simulink model "APFC_FullModel_v23_NoALPF_NodqLPF"  (R2025b)
settings: Solver=ode23t  StartTime=0.0  StopTime=50  MaxStep=2e-4  RelTol=1e-3
undefined symbols (not defined in the file): ALPF_fs, C_B1, C_B2, C_B3, DiscIntNeverNeededParam, FLC_deadband_kVAR, L_B1, L_B2, L_B3, omega, p, Q_reactor, Rc, tau_Qload, X1
libraries: ee_lib x63, fl_lib x59, nesl_utility x43, dspswit3 x9, eeTransforms x2, fuzblock x1, eeSinusoidalMeasurementV2 x1
(part 2 of 4)

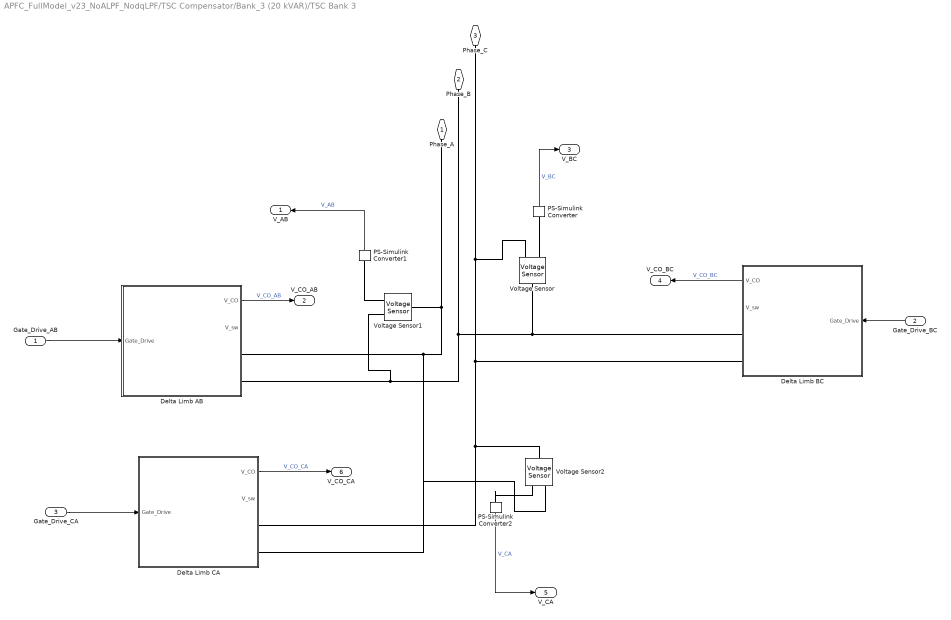
== system APFC_FullModel_v23_NoALPF_NodqLPF/TSC Compensator/Bank_3 (20 kVAR)/TSC Bank 3 ==
  Gate_Drive_AB : Inport
  Gate_Drive_BC : Inport  Port=2
  Gate_Drive_CA : Inport  Port=3
  Delta Limb AB : Subsystem  mask{C_val=C_B3, L_val=L_B3, Rd_val=100e3}
      mask prompts: C_val "Capacitance (F)"; L_val "Inductance (H)"; Rd_val "Discharge Resistance (Ohm)"
      mask help:
      | Delta limb of a three-phase delta-connected TSC bank.
      | Contains: anti-parallel thyristor pair, detuning reactor (L_val,
      | R_series = omega*L_val/Q_reactor), shunt capacitor (C_val), parallel discharge
      | resistor (Rd_val), RC snubber (100 Ohm, 0.1 uF).
      |
      | Output signals:
      | V_sw: instantaneous voltage across the anti-parallel thyristor pair.
      | Used as a diagnostic signal to verify transient-free switching.
      | At the moment of firing, V_sw should be at or near zero. After
      | turn-off, V_sw reflects the difference between the line-to-line
      | source voltage and the capacitor voltage V_C0.
      |
      | V_C0: instantaneous voltage across the shunt capacitor. Fed
      | externally to the ZCD comparator as the residual capacitor voltage
      | reference for voltage-matched firing on subsequent switching events.
      |
      | ZCD logic and gate drive signals are external to this subsystem.
      | Default values correspond to Bank 3 (20 kVAR) at 415 V / 50 Hz
      | with 6% detuning factor. Parameter values for Bank 1 (5 kVAR) and
      | Bank 2 (10 kVAR) are assigned by editing the mask dialog at
      | instantiation.
  Delta Limb BC : Subsystem  mask{C_val=C_B3, L_val=L_B3, Rd_val=100e3}
      mask prompts: C_val "Capacitance (F)"; L_val "Inductance (H)"; Rd_val "Discharge Resistance (Ohm)"
      mask help:
      | Delta limb of a three-phase delta-connected TSC bank.
      | Contains: anti-parallel thyristor pair, detuning reactor (L_val,
      | R_series = omega*L_val/Q_reactor), shunt capacitor (C_val), parallel discharge
      | resistor (Rd_val), RC snubber (100 Ohm, 0.1 uF).
      |
      | Output signals:
      | V_sw: instantaneous voltage across the anti-parallel thyristor pair.
      | Used as a diagnostic signal to verify transient-free switching.
      | At the moment of firing, V_sw should be at or near zero. After
      | turn-off, V_sw reflects the difference between the line-to-line
      | source voltage and the capacitor voltage V_C0.
      |
      | V_C0: instantaneous voltage across the shunt capacitor. Fed
      | externally to the ZCD comparator as the residual capacitor voltage
      | reference for voltage-matched firing on subsequent switching events.
      |
      | ZCD logic and gate drive signals are external to this subsystem.
      | Default values correspond to Bank 3 (20 kVAR) at 415 V / 50 Hz
      | with 6% detuning factor. Parameter values for Bank 1 (5 kVAR) and
      | Bank 2 (10 kVAR) are assigned by editing the mask dialog at
      | instantiation.
  Delta Limb CA : Subsystem  mask{C_val=C_B3, L_val=L_B3, Rd_val=100e3}
      mask prompts: C_val "Capacitance (F)"; L_val "Inductance (H)"; Rd_val "Discharge Resistance (Ohm)"
      mask help:
      | Delta limb of a three-phase delta-connected TSC bank.
      | Contains: anti-parallel thyristor pair, detuning reactor (L_val,
      | R_series = omega*L_val/Q_reactor), shunt capacitor (C_val), parallel discharge
      | resistor (Rd_val), RC snubber (100 Ohm, 0.1 uF).
      |
      | Output signals:
      | V_sw: instantaneous voltage across the anti-parallel thyristor pair.
      | Used as a diagnostic signal to verify transient-free switching.
      | At the moment of firing, V_sw should be at or near zero. After
      | turn-off, V_sw reflects the difference between the line-to-line
      | source voltage and the capacitor voltage V_C0.
      |
      | V_C0: instantaneous voltage across the shunt capacitor. Fed
      | externally to the ZCD comparator as the residual capacitor voltage
      | reference for voltage-matched firing on subsequent switching events.
      |
      | ZCD logic and gate drive signals are external to this subsystem.
      | Default values correspond to Bank 3 (20 kVAR) at 415 V / 50 Hz
      | with 6% detuning factor. Parameter values for Bank 1 (5 kVAR) and
      | Bank 2 (10 kVAR) are assigned by editing the mask dialog at
      | instantiation.
  PS-Simulink Converter : nesl_utility/PS-Simulink Converter  PhysicalDomain=network_engine_domain  SubClassName=ps_output  LeftPortType=input  RightPortType=output  PseudoPeriodic=off  Frequencies=[]  VectorFormat=inherit  Unit=inherit  AffineConversion=off
  PS-Simulink Converter1 : nesl_utility/PS-Simulink Converter  PhysicalDomain=network_engine_domain  SubClassName=ps_output  LeftPortType=input  RightPortType=output  PseudoPeriodic=off  Frequencies=[]  VectorFormat=inherit  Unit=inherit  AffineConversion=off
  PS-Simulink Converter2 : nesl_utility/PS-Simulink Converter  PhysicalDomain=network_engine_domain  SubClassName=ps_output  LeftPortType=input  RightPortType=output  PseudoPeriodic=off  Frequencies=[]  VectorFormat=inherit  Unit=inherit  AffineConversion=off
  Voltage Sensor : fl_lib/Electrical/Electrical Sensors/Voltage Sensor
  Voltage Sensor1 : fl_lib/Electrical/Electrical Sensors/Voltage Sensor
  Voltage Sensor2 : fl_lib/Electrical/Electrical Sensors/Voltage Sensor
  Phase_A : PMIOPort  Side=Left
  Phase_B : PMIOPort  Port=2  Side=Left
  Phase_C : PMIOPort  Port=3  Side=Left
  V_AB : Outport
  V_CO_AB : Outport  Port=2
  V_BC : Outport  Port=3
  V_CO_BC : Outport  Port=4
  V_CA : Outport  Port=5
  V_CO_CA : Outport  Port=6
  wires:
  Delta Limb BC/1(V_CO) -> V_CO_BC/1  "V_CO_BC"
  PS-Simulink Converter/1 -> V_BC/1  "V_BC"
  Gate_Drive_CA/1 -> Delta Limb CA/1(Gate_Drive)
  PS-Simulink Converter1/1 -> V_AB/1  "V_AB"
  Delta Limb AB/1(V_CO) -> V_CO_AB/1  "V_CO_AB"
  Delta Limb CA/1(V_CO) -> V_CO_CA/1  "V_CO_CA"
  Gate_Drive_BC/1 -> Delta Limb BC/1(Gate_Drive)
  Gate_Drive_AB/1 -> Delta Limb AB/1(Gate_Drive)
  PS-Simulink Converter2/1 -> V_CA/1  "V_CA"
  connections:
  Delta Limb BC/RConn1 -- Voltage Sensor/LConn1 -- Phase_B/RConn1 -- Voltage Sensor1/RConn2 -- Delta Limb AB/RConn2
  Voltage Sensor1/RConn1 -- PS-Simulink Converter1/LConn1
  PS-Simulink Converter2/LConn1 -- Voltage Sensor2/RConn1
  Voltage Sensor/RConn2 -- Phase_C/RConn1 -- Delta Limb BC/RConn2 -- Voltage Sensor2/LConn1 -- Delta Limb CA/RConn1
  Voltage Sensor/RConn1 -- PS-Simulink Converter/LConn1
  Voltage Sensor1/LConn1 -- Phase_A/RConn1 -- Voltage Sensor2/RConn2 -- Delta Limb CA/RConn2 -- Delta Limb AB/RConn1

== system APFC_FullModel_v23_NoALPF_NodqLPF/TSC Compensator/Bank_3 (20 kVAR)/ZCD Bank 3 ==
  V_AB : Inport
  V_CO_AB : Inport  Port=2
  V_BC : Inport  Port=3
  V_CO_BC : Inport  Port=4
  V_CA : Inport  Port=5
  V_CO_CA : Inport  Port=6
  Enable : Inport  Port=7
  ZCD AB : Subsystem
      mask help:
      | Zero-Crossing Detection (ZCD) subsystem for one delta limb of a
      | three-phase delta-connected TSC bank.
      |
      | Implements voltage-matched firing logic for transient-free
      | thyristor switching.
      |
      | Inputs:
      | V_source: instantaneous line-to-line voltage for this limb,
      | fed through a Unit Delay (T_s = 0.0001 s) to the comparator.
      |
      | V_C0: residual capacitor voltage from the corresponding
      | Delta_Limb instance, fed through a Unit Delay (T_s = 0.0001 s)
      | to the comparator.
      |
      | Enable: FLC switching command (S = 1 to arm, S = 0 to inhibit).
      | Set to Constant = 1 for open-loop testing.
      |
      | Output:
      | Gate_drive: firing pulse issued when V_source >= V_C0 on a
      | rising edge, AND Enable = 1. Fed to the Gate_drive inport of
      | the corresponding Delta_Limb instance.
      |
      | Internal blocks: Unit Delay (x2), Relational Operator (>=),
      | Zero-Order Hold (T_s = 0.0001 s), Edge Detector (rising edge),
      | AND gate.
      |
      | One instance required per delta limb: ZCD_AB, ZCD_BC, ZCD_CA.
  ZCD BC : Subsystem
      mask help:
      | Zero-Crossing Detection (ZCD) subsystem for one delta limb of a
      | three-phase delta-connected TSC bank.
      |
      | Implements voltage-matched firing logic for transient-free
      | thyristor switching.
      |
      | Inputs:
      | V_source: instantaneous line-to-line voltage for this limb,
      | fed through a Unit Delay (T_s = 0.0001 s) to the comparator.
      |
      | V_C0: residual capacitor voltage from the corresponding
      | Delta_Limb instance, fed through a Unit Delay (T_s = 0.0001 s)
      | to the comparator.
      |
      | Enable: FLC switching command (S = 1 to arm, S = 0 to inhibit).
      | Set to Constant = 1 for open-loop testing.
      |
      | Output:
      | Gate_drive: firing pulse issued when V_source >= V_C0 on a
      | rising edge, AND Enable = 1. Fed to the Gate_drive inport of
      | the corresponding Delta_Limb instance.
      |
      | Internal blocks: Unit Delay (x2), Relational Operator (>=),
      | Zero-Order Hold (T_s = 0.0001 s), Edge Detector (rising edge),
      | AND gate.
      |
      | One instance required per delta limb: ZCD_AB, ZCD_BC, ZCD_CA.
  ZCD CA : Subsystem
      mask help:
      | Zero-Crossing Detection (ZCD) subsystem for one delta limb of a
      | three-phase delta-connected TSC bank.
      |
      | Implements voltage-matched firing logic for transient-free
      | thyristor switching.
      |
      | Inputs:
      | V_source: instantaneous line-to-line voltage for this limb,
      | fed through a Unit Delay (T_s = 0.0001 s) to the comparator.
      |
      | V_C0: residual capacitor voltage from the corresponding
      | Delta_Limb instance, fed through a Unit Delay (T_s = 0.0001 s)
      | to the comparator.
      |
      | Enable: FLC switching command (S = 1 to arm, S = 0 to inhibit).
      | Set to Constant = 1 for open-loop testing.
      |
      | Output:
      | Gate_drive: firing pulse issued when V_source >= V_C0 on a
      | rising edge, AND Enable = 1. Fed to the Gate_drive inport of
      | the corresponding Delta_Limb instance.
      |
      | Internal blocks: Unit Delay (x2), Relational Operator (>=),
      | Zero-Order Hold (T_s = 0.0001 s), Edge Detector (rising edge),
      | AND gate.
      |
      | One instance required per delta limb: ZCD_AB, ZCD_BC, ZCD_CA.
  Gate_drive_AB : Outport
  Gate_drive_BC : Outport  Port=2
  Gate_drive_CA : Outport  Port=3
  wires:
  V_BC/1 -> ZCD BC/2(V_BC)
  Enable/1 -> ZCD AB/3(Enable), ZCD CA/3(Enable), ZCD BC/3(Enable)
  V_CO_BC/1 -> ZCD BC/1(V_CO_BC)
  V_CA/1 -> ZCD CA/2(V_CA)
  V_AB/1 -> ZCD AB/2(V_AB)
  ZCD BC/1(Gate_drive_BC) -> Gate_drive_BC/1
  V_CO_CA/1 -> ZCD CA/1(V_CO_CA)
  ZCD AB/1(Gate_drive_AB) -> Gate_drive_AB/1
  V_CO_AB/1 -> ZCD AB/1(V_CO_AB)
  ZCD CA/1(Gate_drive_CA) -> Gate_drive_CA/1

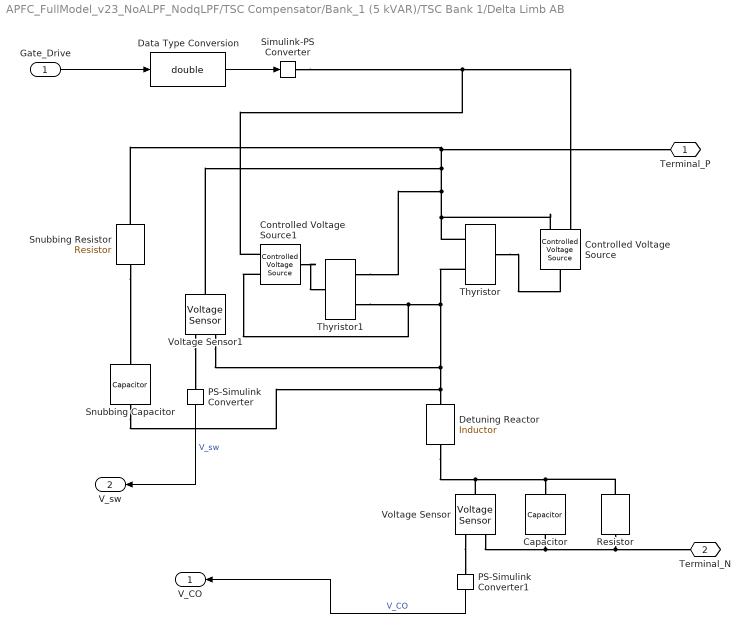
== system APFC_FullModel_v23_NoALPF_NodqLPF/TSC Compensator/Bank_1 (5 kVAR)/TSC Bank 1/Delta Limb AB ==
  Gate_Drive : Inport
  Capacitor : ee_lib/Passive/Capacitor  cap_option=ee.enum.passive.capacitor.capOption.const  c=C_val F  Cvec=[1e-05, 1e-06] F  Vvec=[0, 10] V  CV_table_symmetry=ee.enum.passive.capacitor.tableSymmetry.yes  f_vec=[1, 10] kHz  DFext_vec=[.8, 1.2]  enable_C_tol=ee.enum.toleranceApplication.none  averaging_period=0 s  C_tol=5  tol_distribution=ee.enum.toleranceDistribution.uniform  nSigma=4  r=0 Ohm  g=0 1/Ohm  enable_operating_limits=ee.enum.enable.no  operating_limit_action=ee.enum.passive.reportOpLim.warn  max_working_voltage_range=[-25, 25] V  power_rating=1 W  maxTemperature=85 degC  thermalEnable=false  thermalMass=1 J/K  i_specify=off  i_priority=None  i=0 A  i_nominal_specify=off  i_nominal_value=1  i_nominal_unit=A  v_specify=on  v_priority=High  v=0 V  v_nominal_specify=off  v_nominal_value=1  v_nominal_unit=V  vc_specify=off  vc_priority=High  vc=0 V  vc_nominal_specify=off  vc_nominal_value=1  vc_nominal_unit=V  T_specify=off  T_priority=None  T=298.15 K  T_nominal_specify=off  T_nominal_value=1  T_nominal_unit=K
  Controlled Voltage Source : fl_lib/Electrical/Electrical Sources/Controlled Voltage Source
  Controlled Voltage Source1 : fl_lib/Electrical/Electrical Sources/Controlled Voltage Source
  Data Type Conversion : DataTypeConversion  OutDataTypeStr=double  SaturateOnIntegerOverflow=off  RndMeth=Floor
  Detuning Reactor : ee_lib/Passive/Inductor  l=L_val H  enable_L_tol=ee.enum.toleranceApplication.none  L_tol=20  tol_distribution=ee.enum.toleranceDistribution.uniform  nSigma=4  r=omega*L_val/Q_reactor Ohm  g=1e-9 1/Ohm  enable_operating_limits=ee.enum.enable.no  operating_limit_action=ee.enum.passive.reportOpLim.warn  max_working_current=1 A  power_rating=1 W  i_L_specify=off  i_L_priority=High  i_L=0 A  i_L_nominal_specify=off  i_L_nominal_value=1  i_L_nominal_unit=A
  PS-Simulink Converter : nesl_utility/PS-Simulink Converter  PhysicalDomain=network_engine_domain  SubClassName=ps_output  LeftPortType=input  RightPortType=output  PseudoPeriodic=off  Frequencies=[]  VectorFormat=inherit  Unit=inherit  AffineConversion=off
  PS-Simulink Converter1 : nesl_utility/PS-Simulink Converter  PhysicalDomain=network_engine_domain  SubClassName=ps_output  LeftPortType=input  RightPortType=output  PseudoPeriodic=off  Frequencies=[]  VectorFormat=inherit  Unit=inherit  AffineConversion=off
  Resistor : ee_lib/Passive/Resistor  R=Rd_val Ohm  enable_R_tol=ee.enum.toleranceApplication.none  R_tol=5  tol_distribution=ee.enum.toleranceDistribution.uniform  nSigma=4  enable_operating_limits=ee.enum.enable.no  operating_limit_action=ee.enum.passive.reportOpLim.warn  power_rating=1 W  max_working_voltage=100 V  noise_mode=ee.enum.sources.noise.Disabled  Tdevice=25 degC  sample_time=1e-3 s  repeatability=ee.enum.ic.repeatability.notRepeatable  user_seed=0  auto_seed=3402504572  power_derating_T1=70 degC  power_derating_T2=155 degC  operating_temperature_range_vec=[-50, 150] degC  alpha=3.93e-3 1/K  Tmeas=25 degC  thermal_mass=100 J/K  temperature_specify=off  temperature_priority=High  temperature=298.15 K  temperature_nominal_specify=off  temperature_nominal_value=1  temperature_nominal_unit=K
  Simulink-PS Converter : nesl_utility/Simulink-PS Converter  PhysicalDomain=network_engine_domain  SubClassName=ps_input  LeftPortType=input  RightPortType=output  PseudoPeriodic=off  Frequencies=[]  NoiseDistribution=none  NoiseParameters=[]  Unit=1  AffineConversion=off  FilteringAndDerivatives=provide  SimscapeFilterOrder=1  InputFilterTimeConstant=0.001  UdotUserProvided=0
  Snubbing Capacitor : fl_lib/Electrical/Electrical Elements/Capacitor  c=0.1 uF  r=1e-6 Ohm  g=0 1/Ohm  i_specify=off  i_priority=None  i=0 A  i_nominal_specify=off  i_nominal_value=1  i_nominal_unit=A  v_specify=off  v_priority=None  v=0 V  v_nominal_specify=off  v_nominal_value=1  v_nominal_unit=V  vc_specify=off  vc_priority=High  vc=0 V  vc_nominal_specify=off  vc_nominal_value=1  vc_nominal_unit=V
  Snubbing Resistor : ee_lib/Passive/Resistor  R=100 Ohm  enable_R_tol=ee.enum.toleranceApplication.none  R_tol=5  tol_distribution=ee.enum.toleranceDistribution.uniform  nSigma=4  enable_operating_limits=ee.enum.enable.no  operating_limit_action=ee.enum.passive.reportOpLim.warn  power_rating=1 W  max_working_voltage=100 V  noise_mode=ee.enum.sources.noise.Disabled  Tdevice=25 degC  sample_time=1e-3 s  repeatability=ee.enum.ic.repeatability.notRepeatable  user_seed=0  auto_seed=4120988592  power_derating_T1=70 degC  power_derating_T2=155 degC  operating_temperature_range_vec=[-50, 150] degC  alpha=3.93e-3 1/K  Tmeas=25 degC  thermal_mass=100 J/K  temperature_specify=off  temperature_priority=High  temperature=298.15 K  temperature_nominal_specify=off  temperature_nominal_value=1  temperature_nominal_unit=K
  Thyristor : ee_lib/Semiconductors & Converters/Thyristor  model_type=ee.enum.semiconductors.thyristorModelType.tabulated  v_on=1.2 V  i_on=1 A  VT_vec=[.75, 1, 1.25, 1.5, 1.75, 2, 2.25] V  IT_vec=[.015, .22, .75, 1.4, 2, 2.75, 3.45] A  IDRM=0.01 mA  VDRM=600 V  i_H=1 mA  Tmeas=25 degC  i_GT=3 uA  v_GT=0.6 V  V_D=12 V  R=120 Ohm  dVdt=150 V/us  R_GK=1000 Ohm  TF_NPN_parameterization=1  T_d=2 us  i_d=10 mA  TF_NPN=0.3 us  TF_PNP_parameterization=1  TF_PNP=0.3 us  t_on_delay=0 s  t_on_curr=1 mA  t_on_rise=0 s  Rs=87 kOhm  Rgate=10 Ohm  Gain=10  ig_specify=off  ig_priority=None  ig=0 A  ig_nominal_specify=off  ig_nominal_value=1  ig_nominal_unit=A  ia_specify=off  ia_priority=None  ia=0 A  ia_nominal_specify=off  ia_nominal_value=1  ia_nominal_unit=A  vgk_specify=off  vgk_priority=None  vgk=0 V  vgk_nominal_specify=off  vgk_nominal_value=1  vgk_nominal_unit=V  vak_specify=off  vak_priority=None  vak=0 V  vak_nominal_specify=off  vak_nominal_value=1  vak_nominal_unit=V  Q_npn_bc_specify=off  Q_npn_bc_priority=High  Q_npn_bc=0 C  Q_npn_bc_nominal_specify=off  Q_npn_bc_nominal_value=1  Q_npn_bc_nominal_unit=uC  Q_npn_be_specify=off  Q_npn_be_priority=High  Q_npn_be=0 C  Q_npn_be_nominal_specify=off  Q_npn_be_nominal_value=1  Q_npn_be_nominal_unit=uC  Q_pnp_be_specify=off  Q_pnp_be_priority=High  Q_pnp_be=0 C  Q_pnp_be_nominal_specify=off  Q_pnp_be_nominal_value=1  Q_pnp_be_nominal_unit=uC  thermal_network_parameterization=ee.enum.thermalNetworkTopology.junctionCase  Rth=[0, 10] K/W  Rth_Cauer=[1, 3, 10] K/W  Rth_Foster=[.08, .14, .22, .16] K/W  thermal_mass_parameterization=ee.enum.thermalNetwork.timeconstant  thermal_mass=[0, 1] J/K  thermal_mass_Cauer=[.1, .3, 1] J/K  thermal_mass_Foster=[.001, .005, .05, .5] J/K  thermal_time_constant=[0, 10] s  thermal_time_constant_Cauer=[1, 3, 10] s  thermal_time_constant_Foster=[7e-05, .0007, .01, .08] s  thermal_mass_initial_temperatures=[25, 25] degC  thermal_mass_initial_temperatures_Cauer=[25, 25, 25] degC  Tvec_initial_Foster=[25, 25, 25, 25] degC
      settings: InternalSimscapePortConfiguration="{\"Bottom\":[],\"Left\":[{\"id\":\"G\",\"label\":\"\",\"type\":\"foundation.electrical.electrical\"}],\"Right\":[{\"id\":\"A\",\"label\":\"\",\"type\":\"foundation.electrical.electrical\"},{\"id\":\"K\",\"label\":\"\",\"type\":\"foundation.electrical.electrical\"}],\"Top\":[]}"
  Thyristor1 : ee_lib/Semiconductors & Converters/Thyristor  model_type=ee.enum.semiconductors.thyristorModelType.tabulated  v_on=1.2 V  i_on=1 A  VT_vec=[.75, 1, 1.25, 1.5, 1.75, 2, 2.25] V  IT_vec=[.015, .22, .75, 1.4, 2, 2.75, 3.45] A  IDRM=0.01 mA  VDRM=600 V  i_H=1 mA  Tmeas=25 degC  i_GT=3 uA  v_GT=0.6 V  V_D=12 V  R=120 Ohm  dVdt=150 V/us  R_GK=1000 Ohm  TF_NPN_parameterization=1  T_d=2 us  i_d=10 mA  TF_NPN=0.3 us  TF_PNP_parameterization=1  TF_PNP=0.3 us  t_on_delay=0 s  t_on_curr=1 mA  t_on_rise=0 s  Rs=87 kOhm  Rgate=10 Ohm  Gain=10  ig_specify=off  ig_priority=None  ig=0 A  ig_nominal_specify=off  ig_nominal_value=1  ig_nominal_unit=A  ia_specify=off  ia_priority=None  ia=0 A  ia_nominal_specify=off  ia_nominal_value=1  ia_nominal_unit=A  vgk_specify=off  vgk_priority=None  vgk=0 V  vgk_nominal_specify=off  vgk_nominal_value=1  vgk_nominal_unit=V  vak_specify=off  vak_priority=None  vak=0 V  vak_nominal_specify=off  vak_nominal_value=1  vak_nominal_unit=V  Q_npn_bc_specify=off  Q_npn_bc_priority=High  Q_npn_bc=0 C  Q_npn_bc_nominal_specify=off  Q_npn_bc_nominal_value=1  Q_npn_bc_nominal_unit=uC  Q_npn_be_specify=off  Q_npn_be_priority=High  Q_npn_be=0 C  Q_npn_be_nominal_specify=off  Q_npn_be_nominal_value=1  Q_npn_be_nominal_unit=uC  Q_pnp_be_specify=off  Q_pnp_be_priority=High  Q_pnp_be=0 C  Q_pnp_be_nominal_specify=off  Q_pnp_be_nominal_value=1  Q_pnp_be_nominal_unit=uC  thermal_network_parameterization=ee.enum.thermalNetworkTopology.junctionCase  Rth=[0, 10] K/W  Rth_Cauer=[1, 3, 10] K/W  Rth_Foster=[.08, .14, .22, .16] K/W  thermal_mass_parameterization=ee.enum.thermalNetwork.timeconstant  thermal_mass=[0, 1] J/K  thermal_mass_Cauer=[.1, .3, 1] J/K  thermal_mass_Foster=[.001, .005, .05, .5] J/K  thermal_time_constant=[0, 10] s  thermal_time_constant_Cauer=[1, 3, 10] s  thermal_time_constant_Foster=[7e-05, .0007, .01, .08] s  thermal_mass_initial_temperatures=[25, 25] degC  thermal_mass_initial_temperatures_Cauer=[25, 25, 25] degC  Tvec_initial_Foster=[25, 25, 25, 25] degC
      settings: InternalSimscapePortConfiguration="{\"Bottom\":[],\"Left\":[{\"id\":\"G\",\"label\":\"\",\"type\":\"foundation.electrical.electrical\"}],\"Right\":[{\"id\":\"A\",\"label\":\"\",\"type\":\"foundation.electrical.electrical\"},{\"id\":\"K\",\"label\":\"\",\"type\":\"foundation.electrical.electrical\"}],\"Top\":[]}"
  Voltage Sensor : fl_lib/Electrical/Electrical Sensors/Voltage Sensor
  Voltage Sensor1 : fl_lib/Electrical/Electrical Sensors/Voltage Sensor
  Terminal_P : PMIOPort  Side=Right
  Terminal_N : PMIOPort  Port=2  Side=Right
  V_CO : Outport  VectorParamsAs1DForOutWhenUnconnected=off
  V_sw : Outport  Port=2  VectorParamsAs1DForOutWhenUnconnected=off
  wires:
  Data Type Conversion/1 -> Simulink-PS Converter/1
  PS-Simulink Converter1/1 -> V_CO/1  "V_CO"
  PS-Simulink Converter/1 -> V_sw/1  "V_sw"
  Gate_Drive/1 -> Data Type Conversion/1
  connections:
  Controlled Voltage Source1/LConn1 -- Thyristor1/LConn1
  Thyristor/RConn2 -- Controlled Voltage Source/RConn2 -- Thyristor1/RConn1 -- Voltage Sensor1/LConn1 -- Snubbing Resistor/LConn1 -- Terminal_P/RConn1
  Capacitor/LConn1 -- Detuning Reactor/RConn1 -- Voltage Sensor/LConn1 -- Resistor/LConn1
  Snubbing Resistor/RConn1 -- Snubbing Capacitor/LConn1
  Simulink-PS Converter/RConn1 -- Controlled Voltage Source1/RConn1 -- Controlled Voltage Source/RConn1
  Thyristor/RConn1 -- Controlled Voltage Source1/RConn2 -- Thyristor1/RConn2 -- Voltage Sensor1/RConn2 -- Snubbing Capacitor/RConn1 -- Detuning Reactor/LConn1
  Voltage Sensor/RConn1 -- PS-Simulink Converter1/LConn1
  Voltage Sensor/RConn2 -- Capacitor/RConn1 -- Terminal_N/RConn1 -- Resistor/RConn1
  Thyristor/LConn1 -- Controlled Voltage Source/LConn1
  Voltage Sensor1/RConn1 -- PS-Simulink Converter/LConn1

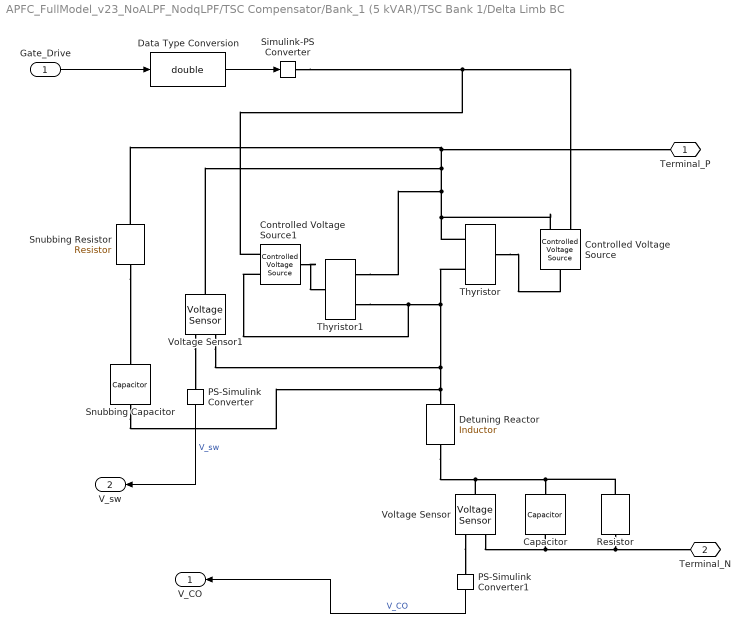
== system APFC_FullModel_v23_NoALPF_NodqLPF/TSC Compensator/Bank_1 (5 kVAR)/TSC Bank 1/Delta Limb BC ==
  Gate_Drive : Inport
  Capacitor : ee_lib/Passive/Capacitor  cap_option=ee.enum.passive.capacitor.capOption.const  c=C_val F  Cvec=[1e-05, 1e-06] F  Vvec=[0, 10] V  CV_table_symmetry=ee.enum.passive.capacitor.tableSymmetry.yes  f_vec=[1, 10] kHz  DFext_vec=[.8, 1.2]  enable_C_tol=ee.enum.toleranceApplication.none  averaging_period=0 s  C_tol=5  tol_distribution=ee.enum.toleranceDistribution.uniform  nSigma=4  r=0 Ohm  g=0 1/Ohm  enable_operating_limits=ee.enum.enable.no  operating_limit_action=ee.enum.passive.reportOpLim.warn  max_working_voltage_range=[-25, 25] V  power_rating=1 W  maxTemperature=85 degC  thermalEnable=false  thermalMass=1 J/K  i_specify=off  i_priority=None  i=0 A  i_nominal_specify=off  i_nominal_value=1  i_nominal_unit=A  v_specify=on  v_priority=High  v=0 V  v_nominal_specify=off  v_nominal_value=1  v_nominal_unit=V  vc_specify=off  vc_priority=High  vc=0 V  vc_nominal_specify=off  vc_nominal_value=1  vc_nominal_unit=V  T_specify=off  T_priority=None  T=298.15 K  T_nominal_specify=off  T_nominal_value=1  T_nominal_unit=K
  Controlled Voltage Source : fl_lib/Electrical/Electrical Sources/Controlled Voltage Source
  Controlled Voltage Source1 : fl_lib/Electrical/Electrical Sources/Controlled Voltage Source
  Data Type Conversion : DataTypeConversion  OutDataTypeStr=double  SaturateOnIntegerOverflow=off  RndMeth=Floor
  Detuning Reactor : ee_lib/Passive/Inductor  l=L_val H  enable_L_tol=ee.enum.toleranceApplication.none  L_tol=20  tol_distribution=ee.enum.toleranceDistribution.uniform  nSigma=4  r=omega*L_val/Q_reactor Ohm  g=1e-9 1/Ohm  enable_operating_limits=ee.enum.enable.no  operating_limit_action=ee.enum.passive.reportOpLim.warn  max_working_current=1 A  power_rating=1 W  i_L_specify=off  i_L_priority=High  i_L=0 A  i_L_nominal_specify=off  i_L_nominal_value=1  i_L_nominal_unit=A
  PS-Simulink Converter : nesl_utility/PS-Simulink Converter  PhysicalDomain=network_engine_domain  SubClassName=ps_output  LeftPortType=input  RightPortType=output  PseudoPeriodic=off  Frequencies=[]  VectorFormat=inherit  Unit=inherit  AffineConversion=off
  PS-Simulink Converter1 : nesl_utility/PS-Simulink Converter  PhysicalDomain=network_engine_domain  SubClassName=ps_output  LeftPortType=input  RightPortType=output  PseudoPeriodic=off  Frequencies=[]  VectorFormat=inherit  Unit=inherit  AffineConversion=off
  Resistor : ee_lib/Passive/Resistor  R=Rd_val Ohm  enable_R_tol=ee.enum.toleranceApplication.none  R_tol=5  tol_distribution=ee.enum.toleranceDistribution.uniform  nSigma=4  enable_operating_limits=ee.enum.enable.no  operating_limit_action=ee.enum.passive.reportOpLim.warn  power_rating=1 W  max_working_voltage=100 V  noise_mode=ee.enum.sources.noise.Disabled  Tdevice=25 degC  sample_time=1e-3 s  repeatability=ee.enum.ic.repeatability.notRepeatable  user_seed=0  auto_seed=2816384857  power_derating_T1=70 degC  power_derating_T2=155 degC  operating_temperature_range_vec=[-50, 150] degC  alpha=3.93e-3 1/K  Tmeas=25 degC  thermal_mass=100 J/K  temperature_specify=off  temperature_priority=High  temperature=298.15 K  temperature_nominal_specify=off  temperature_nominal_value=1  temperature_nominal_unit=K
  Simulink-PS Converter : nesl_utility/Simulink-PS Converter  PhysicalDomain=network_engine_domain  SubClassName=ps_input  LeftPortType=input  RightPortType=output  PseudoPeriodic=off  Frequencies=[]  NoiseDistribution=none  NoiseParameters=[]  Unit=1  AffineConversion=off  FilteringAndDerivatives=provide  SimscapeFilterOrder=1  InputFilterTimeConstant=0.001  UdotUserProvided=0
  Snubbing Capacitor : fl_lib/Electrical/Electrical Elements/Capacitor  c=0.1 uF  r=1e-6 Ohm  g=0 1/Ohm  i_specify=off  i_priority=None  i=0 A  i_nominal_specify=off  i_nominal_value=1  i_nominal_unit=A  v_specify=off  v_priority=None  v=0 V  v_nominal_specify=off  v_nominal_value=1  v_nominal_unit=V  vc_specify=off  vc_priority=High  vc=0 V  vc_nominal_specify=off  vc_nominal_value=1  vc_nominal_unit=V
  Snubbing Resistor : ee_lib/Passive/Resistor  R=100 Ohm  enable_R_tol=ee.enum.toleranceApplication.none  R_tol=5  tol_distribution=ee.enum.toleranceDistribution.uniform  nSigma=4  enable_operating_limits=ee.enum.enable.no  operating_limit_action=ee.enum.passive.reportOpLim.warn  power_rating=1 W  max_working_voltage=100 V  noise_mode=ee.enum.sources.noise.Disabled  Tdevice=25 degC  sample_time=1e-3 s  repeatability=ee.enum.ic.repeatability.notRepeatable  user_seed=0  auto_seed=153380492  power_derating_T1=70 degC  power_derating_T2=155 degC  operating_temperature_range_vec=[-50, 150] degC  alpha=3.93e-3 1/K  Tmeas=25 degC  thermal_mass=100 J/K  temperature_specify=off  temperature_priority=High  temperature=298.15 K  temperature_nominal_specify=off  temperature_nominal_value=1  temperature_nominal_unit=K
  Thyristor : ee_lib/Semiconductors & Converters/Thyristor  model_type=ee.enum.semiconductors.thyristorModelType.tabulated  v_on=1.2 V  i_on=1 A  VT_vec=[.75, 1, 1.25, 1.5, 1.75, 2, 2.25] V  IT_vec=[.015, .22, .75, 1.4, 2, 2.75, 3.45] A  IDRM=0.01 mA  VDRM=600 V  i_H=1 mA  Tmeas=25 degC  i_GT=3 uA  v_GT=0.6 V  V_D=12 V  R=120 Ohm  dVdt=150 V/us  R_GK=1000 Ohm  TF_NPN_parameterization=1  T_d=2 us  i_d=10 mA  TF_NPN=0.3 us  TF_PNP_parameterization=1  TF_PNP=0.3 us  t_on_delay=0 s  t_on_curr=1 mA  t_on_rise=0 s  Rs=87 kOhm  Rgate=10 Ohm  Gain=10  ig_specify=off  ig_priority=None  ig=0 A  ig_nominal_specify=off  ig_nominal_value=1  ig_nominal_unit=A  ia_specify=off  ia_priority=None  ia=0 A  ia_nominal_specify=off  ia_nominal_value=1  ia_nominal_unit=A  vgk_specify=off  vgk_priority=None  vgk=0 V  vgk_nominal_specify=off  vgk_nominal_value=1  vgk_nominal_unit=V  vak_specify=off  vak_priority=None  vak=0 V  vak_nominal_specify=off  vak_nominal_value=1  vak_nominal_unit=V  Q_npn_bc_specify=off  Q_npn_bc_priority=High  Q_npn_bc=0 C  Q_npn_bc_nominal_specify=off  Q_npn_bc_nominal_value=1  Q_npn_bc_nominal_unit=uC  Q_npn_be_specify=off  Q_npn_be_priority=High  Q_npn_be=0 C  Q_npn_be_nominal_specify=off  Q_npn_be_nominal_value=1  Q_npn_be_nominal_unit=uC  Q_pnp_be_specify=off  Q_pnp_be_priority=High  Q_pnp_be=0 C  Q_pnp_be_nominal_specify=off  Q_pnp_be_nominal_value=1  Q_pnp_be_nominal_unit=uC  thermal_network_parameterization=ee.enum.thermalNetworkTopology.junctionCase  Rth=[0, 10] K/W  Rth_Cauer=[1, 3, 10] K/W  Rth_Foster=[.08, .14, .22, .16] K/W  thermal_mass_parameterization=ee.enum.thermalNetwork.timeconstant  thermal_mass=[0, 1] J/K  thermal_mass_Cauer=[.1, .3, 1] J/K  thermal_mass_Foster=[.001, .005, .05, .5] J/K  thermal_time_constant=[0, 10] s  thermal_time_constant_Cauer=[1, 3, 10] s  thermal_time_constant_Foster=[7e-05, .0007, .01, .08] s  thermal_mass_initial_temperatures=[25, 25] degC  thermal_mass_initial_temperatures_Cauer=[25, 25, 25] degC  Tvec_initial_Foster=[25, 25, 25, 25] degC
      settings: InternalSimscapePortConfiguration="{\"Bottom\":[],\"Left\":[{\"id\":\"G\",\"label\":\"\",\"type\":\"foundation.electrical.electrical\"}],\"Right\":[{\"id\":\"A\",\"label\":\"\",\"type\":\"foundation.electrical.electrical\"},{\"id\":\"K\",\"label\":\"\",\"type\":\"foundation.electrical.electrical\"}],\"Top\":[]}"
  Thyristor1 : ee_lib/Semiconductors & Converters/Thyristor  model_type=ee.enum.semiconductors.thyristorModelType.tabulated  v_on=1.2 V  i_on=1 A  VT_vec=[.75, 1, 1.25, 1.5, 1.75, 2, 2.25] V  IT_vec=[.015, .22, .75, 1.4, 2, 2.75, 3.45] A  IDRM=0.01 mA  VDRM=600 V  i_H=1 mA  Tmeas=25 degC  i_GT=3 uA  v_GT=0.6 V  V_D=12 V  R=120 Ohm  dVdt=150 V/us  R_GK=1000 Ohm  TF_NPN_parameterization=1  T_d=2 us  i_d=10 mA  TF_NPN=0.3 us  TF_PNP_parameterization=1  TF_PNP=0.3 us  t_on_delay=0 s  t_on_curr=1 mA  t_on_rise=0 s  Rs=87 kOhm  Rgate=10 Ohm  Gain=10  ig_specify=off  ig_priority=None  ig=0 A  ig_nominal_specify=off  ig_nominal_value=1  ig_nominal_unit=A  ia_specify=off  ia_priority=None  ia=0 A  ia_nominal_specify=off  ia_nominal_value=1  ia_nominal_unit=A  vgk_specify=off  vgk_priority=None  vgk=0 V  vgk_nominal_specify=off  vgk_nominal_value=1  vgk_nominal_unit=V  vak_specify=off  vak_priority=None  vak=0 V  vak_nominal_specify=off  vak_nominal_value=1  vak_nominal_unit=V  Q_npn_bc_specify=off  Q_npn_bc_priority=High  Q_npn_bc=0 C  Q_npn_bc_nominal_specify=off  Q_npn_bc_nominal_value=1  Q_npn_bc_nominal_unit=uC  Q_npn_be_specify=off  Q_npn_be_priority=High  Q_npn_be=0 C  Q_npn_be_nominal_specify=off  Q_npn_be_nominal_value=1  Q_npn_be_nominal_unit=uC  Q_pnp_be_specify=off  Q_pnp_be_priority=High  Q_pnp_be=0 C  Q_pnp_be_nominal_specify=off  Q_pnp_be_nominal_value=1  Q_pnp_be_nominal_unit=uC  thermal_network_parameterization=ee.enum.thermalNetworkTopology.junctionCase  Rth=[0, 10] K/W  Rth_Cauer=[1, 3, 10] K/W  Rth_Foster=[.08, .14, .22, .16] K/W  thermal_mass_parameterization=ee.enum.thermalNetwork.timeconstant  thermal_mass=[0, 1] J/K  thermal_mass_Cauer=[.1, .3, 1] J/K  thermal_mass_Foster=[.001, .005, .05, .5] J/K  thermal_time_constant=[0, 10] s  thermal_time_constant_Cauer=[1, 3, 10] s  thermal_time_constant_Foster=[7e-05, .0007, .01, .08] s  thermal_mass_initial_temperatures=[25, 25] degC  thermal_mass_initial_temperatures_Cauer=[25, 25, 25] degC  Tvec_initial_Foster=[25, 25, 25, 25] degC
      settings: InternalSimscapePortConfiguration="{\"Bottom\":[],\"Left\":[{\"id\":\"G\",\"label\":\"\",\"type\":\"foundation.electrical.electrical\"}],\"Right\":[{\"id\":\"A\",\"label\":\"\",\"type\":\"foundation.electrical.electrical\"},{\"id\":\"K\",\"label\":\"\",\"type\":\"foundation.electrical.electrical\"}],\"Top\":[]}"
  Voltage Sensor : fl_lib/Electrical/Electrical Sensors/Voltage Sensor
  Voltage Sensor1 : fl_lib/Electrical/Electrical Sensors/Voltage Sensor
  Terminal_P : PMIOPort  Side=Right
  Terminal_N : PMIOPort  Port=2  Side=Right
  V_CO : Outport  VectorParamsAs1DForOutWhenUnconnected=off
  V_sw : Outport  Port=2  VectorParamsAs1DForOutWhenUnconnected=off
  wires:
  Data Type Conversion/1 -> Simulink-PS Converter/1
  PS-Simulink Converter1/1 -> V_CO/1  "V_CO"
  PS-Simulink Converter/1 -> V_sw/1  "V_sw"
  Gate_Drive/1 -> Data Type Conversion/1
  connections:
  Controlled Voltage Source1/LConn1 -- Thyristor1/LConn1
  Thyristor/RConn2 -- Controlled Voltage Source/RConn2 -- Thyristor1/RConn1 -- Voltage Sensor1/LConn1 -- Snubbing Resistor/LConn1 -- Terminal_P/RConn1
  Capacitor/LConn1 -- Detuning Reactor/RConn1 -- Voltage Sensor/LConn1 -- Resistor/LConn1
  Snubbing Resistor/RConn1 -- Snubbing Capacitor/LConn1
  Simulink-PS Converter/RConn1 -- Controlled Voltage Source1/RConn1 -- Controlled Voltage Source/RConn1
  Thyristor/RConn1 -- Controlled Voltage Source1/RConn2 -- Thyristor1/RConn2 -- Voltage Sensor1/RConn2 -- Snubbing Capacitor/RConn1 -- Detuning Reactor/LConn1
  Voltage Sensor/RConn1 -- PS-Simulink Converter1/LConn1
  Voltage Sensor/RConn2 -- Capacitor/RConn1 -- Terminal_N/RConn1 -- Resistor/RConn1
  Thyristor/LConn1 -- Controlled Voltage Source/LConn1
  Voltage Sensor1/RConn1 -- PS-Simulink Converter/LConn1

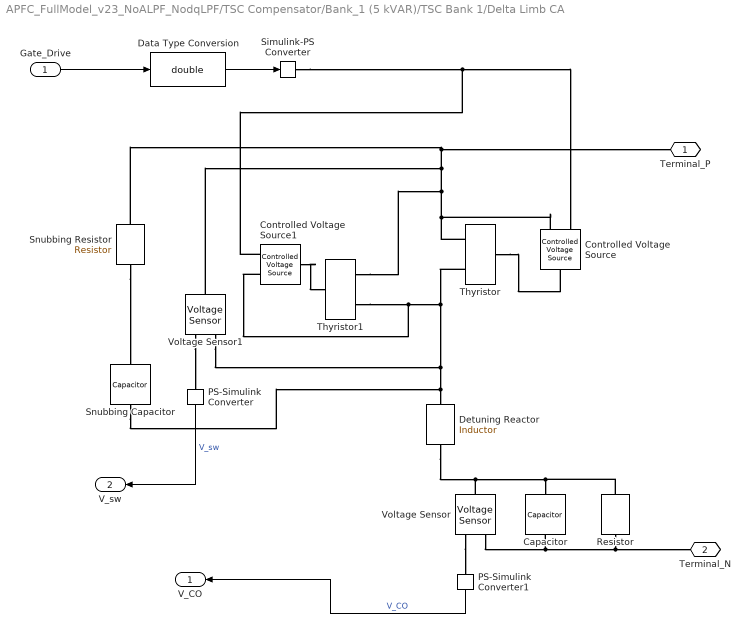
== system APFC_FullModel_v23_NoALPF_NodqLPF/TSC Compensator/Bank_1 (5 kVAR)/TSC Bank 1/Delta Limb CA ==
  Gate_Drive : Inport
  Capacitor : ee_lib/Passive/Capacitor  cap_option=ee.enum.passive.capacitor.capOption.const  c=C_val F  Cvec=[1e-05, 1e-06] F  Vvec=[0, 10] V  CV_table_symmetry=ee.enum.passive.capacitor.tableSymmetry.yes  f_vec=[1, 10] kHz  DFext_vec=[.8, 1.2]  enable_C_tol=ee.enum.toleranceApplication.none  averaging_period=0 s  C_tol=5  tol_distribution=ee.enum.toleranceDistribution.uniform  nSigma=4  r=0 Ohm  g=0 1/Ohm  enable_operating_limits=ee.enum.enable.no  operating_limit_action=ee.enum.passive.reportOpLim.warn  max_working_voltage_range=[-25, 25] V  power_rating=1 W  maxTemperature=85 degC  thermalEnable=false  thermalMass=1 J/K  i_specify=off  i_priority=None  i=0 A  i_nominal_specify=off  i_nominal_value=1  i_nominal_unit=A  v_specify=on  v_priority=High  v=0 V  v_nominal_specify=off  v_nominal_value=1  v_nominal_unit=V  vc_specify=off  vc_priority=High  vc=0 V  vc_nominal_specify=off  vc_nominal_value=1  vc_nominal_unit=V  T_specify=off  T_priority=None  T=298.15 K  T_nominal_specify=off  T_nominal_value=1  T_nominal_unit=K
  Controlled Voltage Source : fl_lib/Electrical/Electrical Sources/Controlled Voltage Source
  Controlled Voltage Source1 : fl_lib/Electrical/Electrical Sources/Controlled Voltage Source
  Data Type Conversion : DataTypeConversion  OutDataTypeStr=double  SaturateOnIntegerOverflow=off  RndMeth=Floor
  Detuning Reactor : ee_lib/Passive/Inductor  l=L_val H  enable_L_tol=ee.enum.toleranceApplication.none  L_tol=20  tol_distribution=ee.enum.toleranceDistribution.uniform  nSigma=4  r=omega*L_val/Q_reactor Ohm  g=1e-9 1/Ohm  enable_operating_limits=ee.enum.enable.no  operating_limit_action=ee.enum.passive.reportOpLim.warn  max_working_current=1 A  power_rating=1 W  i_L_specify=off  i_L_priority=High  i_L=0 A  i_L_nominal_specify=off  i_L_nominal_value=1  i_L_nominal_unit=A
  PS-Simulink Converter : nesl_utility/PS-Simulink Converter  PhysicalDomain=network_engine_domain  SubClassName=ps_output  LeftPortType=input  RightPortType=output  PseudoPeriodic=off  Frequencies=[]  VectorFormat=inherit  Unit=inherit  AffineConversion=off
  PS-Simulink Converter1 : nesl_utility/PS-Simulink Converter  PhysicalDomain=network_engine_domain  SubClassName=ps_output  LeftPortType=input  RightPortType=output  PseudoPeriodic=off  Frequencies=[]  VectorFormat=inherit  Unit=inherit  AffineConversion=off
  Resistor : ee_lib/Passive/Resistor  R=Rd_val Ohm  enable_R_tol=ee.enum.toleranceApplication.none  R_tol=5  tol_distribution=ee.enum.toleranceDistribution.uniform  nSigma=4  enable_operating_limits=ee.enum.enable.no  operating_limit_action=ee.enum.passive.reportOpLim.warn  power_rating=1 W  max_working_voltage=100 V  noise_mode=ee.enum.sources.noise.Disabled  Tdevice=25 degC  sample_time=1e-3 s  repeatability=ee.enum.ic.repeatability.notRepeatable  user_seed=0  auto_seed=3646982598  power_derating_T1=70 degC  power_derating_T2=155 degC  operating_temperature_range_vec=[-50, 150] degC  alpha=3.93e-3 1/K  Tmeas=25 degC  thermal_mass=100 J/K  temperature_specify=off  temperature_priority=High  temperature=298.15 K  temperature_nominal_specify=off  temperature_nominal_value=1  temperature_nominal_unit=K
  Simulink-PS Converter : nesl_utility/Simulink-PS Converter  PhysicalDomain=network_engine_domain  SubClassName=ps_input  LeftPortType=input  RightPortType=output  PseudoPeriodic=off  Frequencies=[]  NoiseDistribution=none  NoiseParameters=[]  Unit=1  AffineConversion=off  FilteringAndDerivatives=provide  SimscapeFilterOrder=1  InputFilterTimeConstant=0.001  UdotUserProvided=0
  Snubbing Capacitor : fl_lib/Electrical/Electrical Elements/Capacitor  c=0.1 uF  r=1e-6 Ohm  g=0 1/Ohm  i_specify=off  i_priority=None  i=0 A  i_nominal_specify=off  i_nominal_value=1  i_nominal_unit=A  v_specify=off  v_priority=None  v=0 V  v_nominal_specify=off  v_nominal_value=1  v_nominal_unit=V  vc_specify=off  vc_priority=High  vc=0 V  vc_nominal_specify=off  vc_nominal_value=1  vc_nominal_unit=V
  Snubbing Resistor : ee_lib/Passive/Resistor  R=100 Ohm  enable_R_tol=ee.enum.toleranceApplication.none  R_tol=5  tol_distribution=ee.enum.toleranceDistribution.uniform  nSigma=4  enable_operating_limits=ee.enum.enable.no  operating_limit_action=ee.enum.passive.reportOpLim.warn  power_rating=1 W  max_working_voltage=100 V  noise_mode=ee.enum.sources.noise.Disabled  Tdevice=25 degC  sample_time=1e-3 s  repeatability=ee.enum.ic.repeatability.notRepeatable  user_seed=0  auto_seed=4011470453  power_derating_T1=70 degC  power_derating_T2=155 degC  operating_temperature_range_vec=[-50, 150] degC  alpha=3.93e-3 1/K  Tmeas=25 degC  thermal_mass=100 J/K  temperature_specify=off  temperature_priority=High  temperature=298.15 K  temperature_nominal_specify=off  temperature_nominal_value=1  temperature_nominal_unit=K
  Thyristor : ee_lib/Semiconductors & Converters/Thyristor  model_type=ee.enum.semiconductors.thyristorModelType.tabulated  v_on=1.2 V  i_on=1 A  VT_vec=[.75, 1, 1.25, 1.5, 1.75, 2, 2.25] V  IT_vec=[.015, .22, .75, 1.4, 2, 2.75, 3.45] A  IDRM=0.01 mA  VDRM=600 V  i_H=1 mA  Tmeas=25 degC  i_GT=3 uA  v_GT=0.6 V  V_D=12 V  R=120 Ohm  dVdt=150 V/us  R_GK=1000 Ohm  TF_NPN_parameterization=1  T_d=2 us  i_d=10 mA  TF_NPN=0.3 us  TF_PNP_parameterization=1  TF_PNP=0.3 us  t_on_delay=0 s  t_on_curr=1 mA  t_on_rise=0 s  Rs=87 kOhm  Rgate=10 Ohm  Gain=10  ig_specify=off  ig_priority=None  ig=0 A  ig_nominal_specify=off  ig_nominal_value=1  ig_nominal_unit=A  ia_specify=off  ia_priority=None  ia=0 A  ia_nominal_specify=off  ia_nominal_value=1  ia_nominal_unit=A  vgk_specify=off  vgk_priority=None  vgk=0 V  vgk_nominal_specify=off  vgk_nominal_value=1  vgk_nominal_unit=V  vak_specify=off  vak_priority=None  vak=0 V  vak_nominal_specify=off  vak_nominal_value=1  vak_nominal_unit=V  Q_npn_bc_specify=off  Q_npn_bc_priority=High  Q_npn_bc=0 C  Q_npn_bc_nominal_specify=off  Q_npn_bc_nominal_value=1  Q_npn_bc_nominal_unit=uC  Q_npn_be_specify=off  Q_npn_be_priority=High  Q_npn_be=0 C  Q_npn_be_nominal_specify=off  Q_npn_be_nominal_value=1  Q_npn_be_nominal_unit=uC  Q_pnp_be_specify=off  Q_pnp_be_priority=High  Q_pnp_be=0 C  Q_pnp_be_nominal_specify=off  Q_pnp_be_nominal_value=1  Q_pnp_be_nominal_unit=uC  thermal_network_parameterization=ee.enum.thermalNetworkTopology.junctionCase  Rth=[0, 10] K/W  Rth_Cauer=[1, 3, 10] K/W  Rth_Foster=[.08, .14, .22, .16] K/W  thermal_mass_parameterization=ee.enum.thermalNetwork.timeconstant  thermal_mass=[0, 1] J/K  thermal_mass_Cauer=[.1, .3, 1] J/K  thermal_mass_Foster=[.001, .005, .05, .5] J/K  thermal_time_constant=[0, 10] s  thermal_time_constant_Cauer=[1, 3, 10] s  thermal_time_constant_Foster=[7e-05, .0007, .01, .08] s  thermal_mass_initial_temperatures=[25, 25] degC  thermal_mass_initial_temperatures_Cauer=[25, 25, 25] degC  Tvec_initial_Foster=[25, 25, 25, 25] degC
      settings: InternalSimscapePortConfiguration="{\"Bottom\":[],\"Left\":[{\"id\":\"G\",\"label\":\"\",\"type\":\"foundation.electrical.electrical\"}],\"Right\":[{\"id\":\"A\",\"label\":\"\",\"type\":\"foundation.electrical.electrical\"},{\"id\":\"K\",\"label\":\"\",\"type\":\"foundation.electrical.electrical\"}],\"Top\":[]}"
  Thyristor1 : ee_lib/Semiconductors & Converters/Thyristor  model_type=ee.enum.semiconductors.thyristorModelType.tabulated  v_on=1.2 V  i_on=1 A  VT_vec=[.75, 1, 1.25, 1.5, 1.75, 2, 2.25] V  IT_vec=[.015, .22, .75, 1.4, 2, 2.75, 3.45] A  IDRM=0.01 mA  VDRM=600 V  i_H=1 mA  Tmeas=25 degC  i_GT=3 uA  v_GT=0.6 V  V_D=12 V  R=120 Ohm  dVdt=150 V/us  R_GK=1000 Ohm  TF_NPN_parameterization=1  T_d=2 us  i_d=10 mA  TF_NPN=0.3 us  TF_PNP_parameterization=1  TF_PNP=0.3 us  t_on_delay=0 s  t_on_curr=1 mA  t_on_rise=0 s  Rs=87 kOhm  Rgate=10 Ohm  Gain=10  ig_specify=off  ig_priority=None  ig=0 A  ig_nominal_specify=off  ig_nominal_value=1  ig_nominal_unit=A  ia_specify=off  ia_priority=None  ia=0 A  ia_nominal_specify=off  ia_nominal_value=1  ia_nominal_unit=A  vgk_specify=off  vgk_priority=None  vgk=0 V  vgk_nominal_specify=off  vgk_nominal_value=1  vgk_nominal_unit=V  vak_specify=off  vak_priority=None  vak=0 V  vak_nominal_specify=off  vak_nominal_value=1  vak_nominal_unit=V  Q_npn_bc_specify=off  Q_npn_bc_priority=High  Q_npn_bc=0 C  Q_npn_bc_nominal_specify=off  Q_npn_bc_nominal_value=1  Q_npn_bc_nominal_unit=uC  Q_npn_be_specify=off  Q_npn_be_priority=High  Q_npn_be=0 C  Q_npn_be_nominal_specify=off  Q_npn_be_nominal_value=1  Q_npn_be_nominal_unit=uC  Q_pnp_be_specify=off  Q_pnp_be_priority=High  Q_pnp_be=0 C  Q_pnp_be_nominal_specify=off  Q_pnp_be_nominal_value=1  Q_pnp_be_nominal_unit=uC  thermal_network_parameterization=ee.enum.thermalNetworkTopology.junctionCase  Rth=[0, 10] K/W  Rth_Cauer=[1, 3, 10] K/W  Rth_Foster=[.08, .14, .22, .16] K/W  thermal_mass_parameterization=ee.enum.thermalNetwork.timeconstant  thermal_mass=[0, 1] J/K  thermal_mass_Cauer=[.1, .3, 1] J/K  thermal_mass_Foster=[.001, .005, .05, .5] J/K  thermal_time_constant=[0, 10] s  thermal_time_constant_Cauer=[1, 3, 10] s  thermal_time_constant_Foster=[7e-05, .0007, .01, .08] s  thermal_mass_initial_temperatures=[25, 25] degC  thermal_mass_initial_temperatures_Cauer=[25, 25, 25] degC  Tvec_initial_Foster=[25, 25, 25, 25] degC
      settings: InternalSimscapePortConfiguration="{\"Bottom\":[],\"Left\":[{\"id\":\"G\",\"label\":\"\",\"type\":\"foundation.electrical.electrical\"}],\"Right\":[{\"id\":\"A\",\"label\":\"\",\"type\":\"foundation.electrical.electrical\"},{\"id\":\"K\",\"label\":\"\",\"type\":\"foundation.electrical.electrical\"}],\"Top\":[]}"
  Voltage Sensor : fl_lib/Electrical/Electrical Sensors/Voltage Sensor
  Voltage Sensor1 : fl_lib/Electrical/Electrical Sensors/Voltage Sensor
  Terminal_P : PMIOPort  Side=Right
  Terminal_N : PMIOPort  Port=2  Side=Right
  V_CO : Outport  VectorParamsAs1DForOutWhenUnconnected=off
  V_sw : Outport  Port=2  VectorParamsAs1DForOutWhenUnconnected=off
  wires:
  Data Type Conversion/1 -> Simulink-PS Converter/1
  PS-Simulink Converter1/1 -> V_CO/1  "V_CO"
  PS-Simulink Converter/1 -> V_sw/1  "V_sw"
  Gate_Drive/1 -> Data Type Conversion/1
  connections:
  Controlled Voltage Source1/LConn1 -- Thyristor1/LConn1
  Thyristor/RConn2 -- Controlled Voltage Source/RConn2 -- Thyristor1/RConn1 -- Voltage Sensor1/LConn1 -- Snubbing Resistor/LConn1 -- Terminal_P/RConn1
  Capacitor/LConn1 -- Detuning Reactor/RConn1 -- Voltage Sensor/LConn1 -- Resistor/LConn1
  Snubbing Resistor/RConn1 -- Snubbing Capacitor/LConn1
  Simulink-PS Converter/RConn1 -- Controlled Voltage Source1/RConn1 -- Controlled Voltage Source/RConn1
  Thyristor/RConn1 -- Controlled Voltage Source1/RConn2 -- Thyristor1/RConn2 -- Voltage Sensor1/RConn2 -- Snubbing Capacitor/RConn1 -- Detuning Reactor/LConn1
  Voltage Sensor/RConn1 -- PS-Simulink Converter1/LConn1
  Voltage Sensor/RConn2 -- Capacitor/RConn1 -- Terminal_N/RConn1 -- Resistor/RConn1
  Thyristor/LConn1 -- Controlled Voltage Source/LConn1
  Voltage Sensor1/RConn1 -- PS-Simulink Converter/LConn1

== system APFC_FullModel_v23_NoALPF_NodqLPF/TSC Compensator/Bank_1 (5 kVAR)/ZCD Bank 1/ZCD AB ==
  V_CO_AB : Inport
  V_AB : Inport  Port=2
  Enable : Inport  Port=3
  AND : Logic  IconShape=distinctive  AllPortsSameDT=off  OutDataTypeStr=boolean
  Edge Detector : dspswit3/Edge Detector  InputProcessing=Columns as channels (frame based)
  OR : Logic  Operator=OR  IconShape=distinctive  AllPortsSameDT=off  OutDataTypeStr=boolean
  Relational Operator : RelationalOperator  OutDataTypeStr=boolean  RndMeth=Simplest  InputSameDT=off
  Unit Delay : UnitDelay  SampleTime=0.0001  HasFrameUpgradeWarning=on
  Unit Delay1 : UnitDelay  SampleTime=0.0001  HasFrameUpgradeWarning=on
  Unit Delay2 : UnitDelay  SampleTime=1e-4  HasFrameUpgradeWarning=on
  Zero-Order Hold : ZeroOrderHold  SampleTime=0.0001
  Gate_drive_AB : Outport
  wires:
  V_CO_AB/1 -> Unit Delay/1
  Unit Delay1/1 -> Relational Operator/1
  Zero-Order Hold/1 -> Edge Detector/1
  Unit Delay/1 -> Relational Operator/2
  Relational Operator/1 -> Zero-Order Hold/1
  V_AB/1 -> Unit Delay1/1
  Enable/1 -> AND/2
  AND/1 -> Unit Delay2/1, Gate_drive_AB/1
  Edge Detector/1 -> OR/1
  OR/1 -> AND/1
  Unit Delay2/1 -> OR/2

== system APFC_FullModel_v23_NoALPF_NodqLPF/TSC Compensator/Bank_1 (5 kVAR)/ZCD Bank 1/ZCD BC ==
  V_CO_BC : Inport
  V_BC : Inport  Port=2
  Enable : Inport  Port=3
  AND : Logic  IconShape=distinctive  AllPortsSameDT=off  OutDataTypeStr=boolean
  Edge Detector : dspswit3/Edge Detector  InputProcessing=Columns as channels (frame based)
  OR : Logic  Operator=OR  IconShape=distinctive  AllPortsSameDT=off  OutDataTypeStr=boolean
  Relational Operator : RelationalOperator  OutDataTypeStr=boolean  RndMeth=Simplest  InputSameDT=off
  Unit Delay : UnitDelay  SampleTime=0.0001  HasFrameUpgradeWarning=on
  Unit Delay1 : UnitDelay  SampleTime=0.0001  HasFrameUpgradeWarning=on
  Unit Delay2 : UnitDelay  SampleTime=-1  HasFrameUpgradeWarning=on
  Zero-Order Hold : ZeroOrderHold  SampleTime=0.0001
  Gate_drive_BC : Outport
  wires:
  V_CO_BC/1 -> Unit Delay/1
  Unit Delay1/1 -> Relational Operator/1
  Zero-Order Hold/1 -> Edge Detector/1
  Unit Delay/1 -> Relational Operator/2
  Relational Operator/1 -> Zero-Order Hold/1
  V_BC/1 -> Unit Delay1/1
  Enable/1 -> AND/2
  AND/1 -> Unit Delay2/1, Gate_drive_BC/1
  OR/1 -> AND/1
  Edge Detector/1 -> OR/1
  Unit Delay2/1 -> OR/2

== system APFC_FullModel_v23_NoALPF_NodqLPF/TSC Compensator/Bank_1 (5 kVAR)/ZCD Bank 1/ZCD CA ==
  V_CO_CA : Inport
  V_CA : Inport  Port=2
  Enable : Inport  Port=3
  AND : Logic  IconShape=distinctive  AllPortsSameDT=off  OutDataTypeStr=boolean
  Edge Detector : dspswit3/Edge Detector  InputProcessing=Columns as channels (frame based)
  OR : Logic  Operator=OR  IconShape=distinctive  AllPortsSameDT=off  OutDataTypeStr=boolean
  Relational Operator : RelationalOperator  OutDataTypeStr=boolean  RndMeth=Simplest  InputSameDT=off
  Unit Delay : UnitDelay  SampleTime=0.0001  HasFrameUpgradeWarning=on
  Unit Delay1 : UnitDelay  SampleTime=0.0001  HasFrameUpgradeWarning=on
  Unit Delay2 : UnitDelay  SampleTime=1e-4  HasFrameUpgradeWarning=on
  Zero-Order Hold : ZeroOrderHold  SampleTime=0.0001
  Gate_drive_CA : Outport
  wires:
  V_CO_CA/1 -> Unit Delay/1
  Unit Delay1/1 -> Relational Operator/1
  Zero-Order Hold/1 -> Edge Detector/1
  Unit Delay/1 -> Relational Operator/2
  Relational Operator/1 -> Zero-Order Hold/1
  V_CA/1 -> Unit Delay1/1
  Enable/1 -> AND/2
  AND/1 -> Unit Delay2/1, Gate_drive_CA/1
  OR/1 -> AND/1
  Edge Detector/1 -> OR/1
  Unit Delay2/1 -> OR/2
